simulink model "Section1_h"  (R2023b)
settings: Solver=VariableStepAuto  StartTime=0.0  StopTime=10.0  RelTol=1e-3
settings Model: Creator=afra  LastModifiedBy=paria

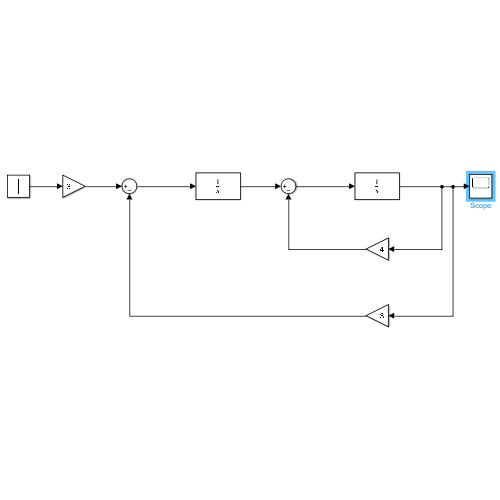
[thumbnail: Simulink's stored preview of the top-level diagram]
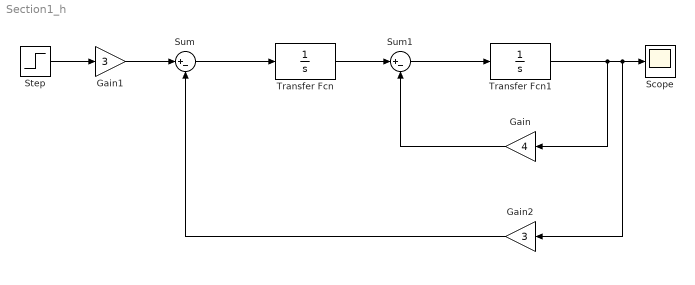
== system Section1_h ==
  Gain : Gain  Gain=4
  Gain1 : Gain  Gain=3
  Gain2 : Gain  Gain=3
  Scope : Scope
  Step : Step  Time=0  SampleTime=0
  Sum : Sum  Inputs=|+-
  Sum1 : Sum  Inputs=|+-
  Transfer Fcn : TransferFcn  Denominator=[1 0]
  Transfer Fcn1 : TransferFcn  Denominator=[1 0]
  wires:
  Step/1 -> Gain1/1
  Gain1/1 -> Sum/1
  Sum/1 -> Transfer Fcn/1
  Transfer Fcn/1 -> Sum1/1
  Sum1/1 -> Transfer Fcn1/1
  Transfer Fcn1/1 -> Gain/1, Gain2/1, Scope/1
  Gain/1 -> Sum1/2
  Gain2/1 -> Sum/2
